simulink model "PF_ToolwithMedusa_Fix"  (R2016a)
settings: Solver=ode45  StartTime=0.0  StopTime=250  FixedStep=Ts  RelTol=1e-3
values from neighbouring files (symbols this model uses):
  Ts = 0.2    [PFtools.m]    (also in RK4_integrator.m = input.Ts; Trajectory_tracking.m = 0.1)
settings Model: Creator=hung  LastModifiedBy=hung
settings DataIOCC: LimitDataPoints=on  SaveFormat=Array
settings DebuggingCC: UnderspecifiedInitializationDetection=Classic  MergeDetectMultiDrivingBlocksExec=none  SolverPrmCheckMsg=warning  StateNameClashWarn=warning
settings HardwareCC: ProdBitPerPointer=32  ProdLargestAtomicFloat=None  ProdIntDivRoundTo=Undefined  ProdEndianess=Unspecified  ProdWordSize=32  ProdHWDeviceType=32-bit Generic
settings ModelReferenceCC: PropagateSignalLabelsOutOfModel=off
settings ConfigComp: CovModelRefEnable=Off

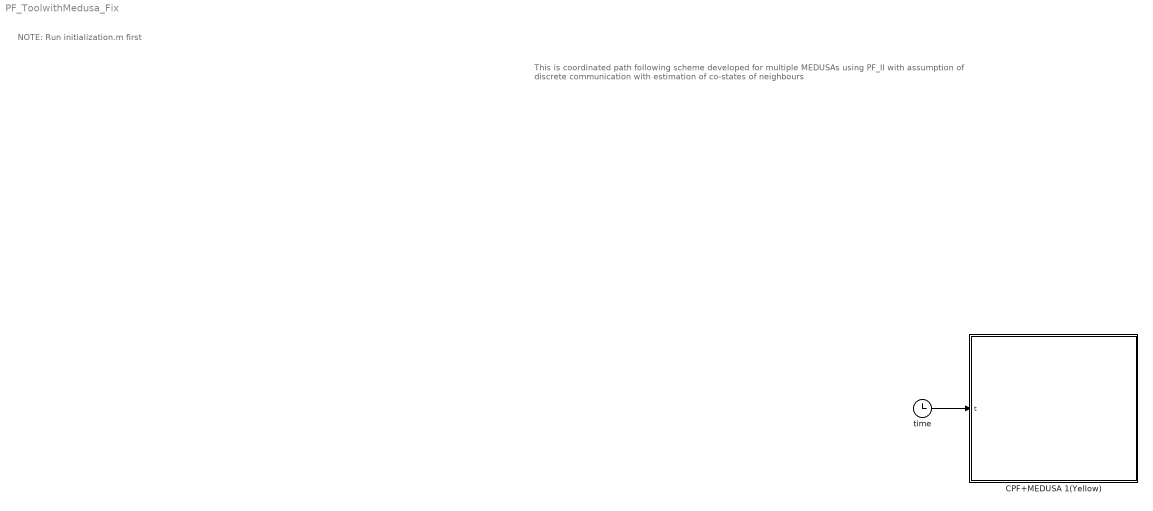
== system PF_ToolwithMedusa_Fix ==
  note: NOTE: Run initialization.m first
  note: This is coordinated path following scheme developed for multiple MEDUSAs using PF_II with
      | assumption of discrete communication with estimation of co-states of neighbours
  CPF+MEDUSA 1(Yellow) : Subsystem  Priority=2  TreatAsAtomicUnit=on  mask{Vehicle_Index=1}
      mask Display: image('MEDUSA_YELLOW.png');
  time : Clock
  wires:
  time/1 -> CPF+MEDUSA 1(Yellow)/1(t)

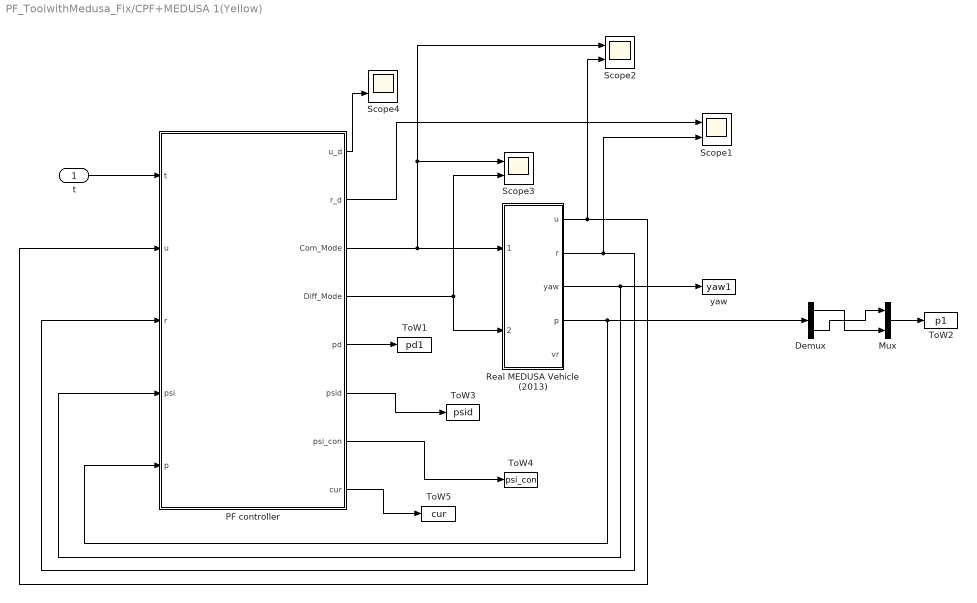
== system PF_ToolwithMedusa_Fix/CPF+MEDUSA 1(Yellow) ==
  t : Inport
  " Real MEDUSA Vehicle (2013)" : Subsystem  AncestorBlock=|
      | Mylibrary/
      | Real MEDUSA Vehicle (2013)
  Demux : Demux  Outputs=2
  Mux : Mux  Inputs=2
  "PF controller " : MATLAB Function  TreatAsAtomicUnit=on
  Scope{1..4} (4 alike) : Scope  NumInputPorts=2
  ToW1 : ToWorkspace  VariableName=pd1  SampleTime=Ts
      settings: Save2DSignal=2-D array (concatenate along first dimension)
  ToW2 : ToWorkspace  VariableName=p1  SampleTime=Ts
  ToW3 : ToWorkspace  VariableName=psid  SampleTime=Ts
      settings: Save2DSignal=2-D array (concatenate along first dimension)
  ToW4 : ToWorkspace  VariableName=psi_con  SampleTime=Ts
      settings: Save2DSignal=2-D array (concatenate along first dimension)
  ToW5 : ToWorkspace  VariableName=cur  SampleTime=Ts
      settings: Save2DSignal=2-D array (concatenate along first dimension)
  yaw : ToWorkspace  VariableName=yaw1  SampleTime=Ts
  wires:
  t/1 -> "PF controller "/1(t)
  "PF controller "/5(pd) -> ToW1/1
  "PF controller "/3(Com_Mode) -> " Real MEDUSA Vehicle (2013)"/1(Com Mode), Scope2/1, Scope3/1
  "PF controller "/2(r_d) -> Scope1/1
  "PF controller "/4(Diff_Mode) -> " Real MEDUSA Vehicle (2013)"/2(Diff Mode), Scope3/2
  " Real MEDUSA Vehicle (2013)"/4(p) -> Demux/1, "PF controller "/5(p)
  " Real MEDUSA Vehicle (2013)"/3(yaw) -> yaw/1, "PF controller "/4(psi)
  " Real MEDUSA Vehicle (2013)"/2(r) -> Scope1/2, "PF controller "/3(r)
  " Real MEDUSA Vehicle (2013)"/1(u) -> Scope2/2, "PF controller "/2(u)
  "PF controller "/6(psid) -> ToW3/1
  "PF controller "/7(psi_con) -> ToW4/1
  Mux/1 -> ToW2/1
  "PF controller "/8(cur) -> ToW5/1
  Demux/1 -> Mux/2
  Demux/2 -> Mux/1
  "PF controller "/1(u_d) -> Scope4/2

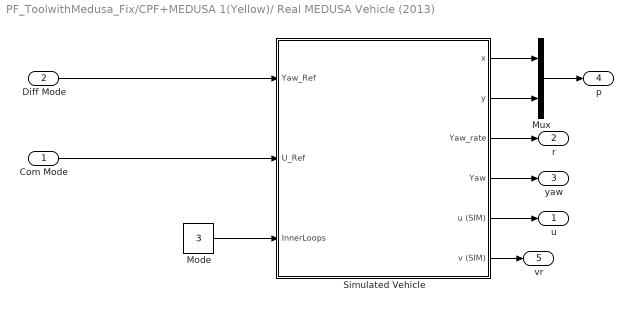
== system PF_ToolwithMedusa_Fix/CPF+MEDUSA 1(Yellow)/ Real MEDUSA Vehicle (2013) ==
  Com Mode : Inport
  Diff Mode : Inport  Port=2
  Mode : Constant  Value=3
  Mux : Mux  Inputs=2
  Simulated Vehicle : Subsystem
  u : Outport
  r : Outport  Port=2
  yaw : Outport  Port=3
  p : Outport  Port=4
  vr : Outport  Port=5
  wires:
  Diff Mode/1 -> Simulated Vehicle/1(Yaw_Ref)
  Com Mode/1 -> Simulated Vehicle/2(U_Ref)
  Mode/1 -> Simulated Vehicle/3(InnerLoops)
  Mux/1 -> p/1
  Simulated Vehicle/5(u (SIM)) -> u/1
  Simulated Vehicle/6(v (SIM)) -> vr/1
  Simulated Vehicle/3(Yaw_rate) -> r/1
  Simulated Vehicle/4(Yaw) -> yaw/1
  Simulated Vehicle/1(x) -> Mux/1
  Simulated Vehicle/2(y) -> Mux/2

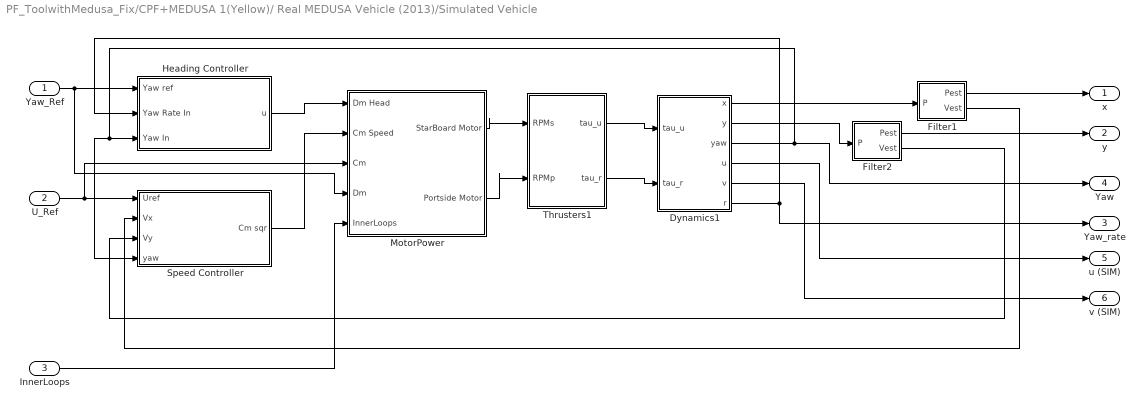
== system PF_ToolwithMedusa_Fix/CPF+MEDUSA 1(Yellow)/ Real MEDUSA Vehicle (2013)/Simulated Vehicle ==
  Yaw_Ref : Inport
  U_Ref : Inport  Port=2
  InnerLoops : Inport  Port=3
  Dynamics1 : Subsystem  mask{x0=200, y0=305, yaw0=pi/2, u0=0, v0=0, r0=0, dist_u=0, dist_v=0, dist_r=0, Vcx=0, Vcy=0}
      mask prompts: dist_u "Disturbance in u"; dist_v "Disturbance in v"; dist_r "Disturbance in r"; Vcx "Current x"; Vcy "Current y"
  Filter1 : Subsystem
  Filter2 : Subsystem
  Heading Controller : Subsystem  mask{Kp=45, Kd=110}
  MotorPower : Subsystem
  "Speed Controller " : Subsystem  mask{Kpu=60, Kiu=2, KSat=60}
      mask prompts: Kpu "Kp"; Kiu "Ki"; KSat "Common Mode Saturation"
  Thrusters1 : Subsystem
  x : Outport
  y : Outport  Port=2
  Yaw_rate : Outport  Port=3
  Yaw : Outport  Port=4
  u (SIM) : Outport  Port=5
  v (SIM) : Outport  Port=6
  wires:
  Thrusters1/1(tau_u) -> Dynamics1/1(tau_u)
  Thrusters1/2(tau_r) -> Dynamics1/2(tau_r)
  Dynamics1/1(x) -> Filter1/1(P)
  Dynamics1/2(y) -> Filter2/1(P)
  Dynamics1/3(yaw) -> Heading Controller/3(Yaw In), "Speed Controller "/4(yaw), Yaw/1
  MotorPower/1(StarBoard Motor) -> Thrusters1/1(RPMs)
  MotorPower/2(Portside Motor) -> Thrusters1/2(RPMp)
  Dynamics1/6(r) -> Heading Controller/2(Yaw Rate In), Yaw_rate/1
  Filter1/2(Vest) -> "Speed Controller "/2(Vx)
  Filter2/2(Vest) -> "Speed Controller "/3(Vy)
  "Speed Controller "/1(Cm sqr) -> MotorPower/2(Cm Speed)
  Yaw_Ref/1 -> Heading Controller/1(Yaw ref), MotorPower/4(Dm)
  Filter1/1(Pest) -> x/1
  Filter2/1(Pest) -> y/1
  U_Ref/1 -> "Speed Controller "/1(Uref), MotorPower/3(Cm)
  Heading Controller/1(u) -> MotorPower/1(Dm Head)
  InnerLoops/1 -> MotorPower/5(InnerLoops)
  Dynamics1/4(u) -> u (SIM)/1
  Dynamics1/5(v) -> v (SIM)/1

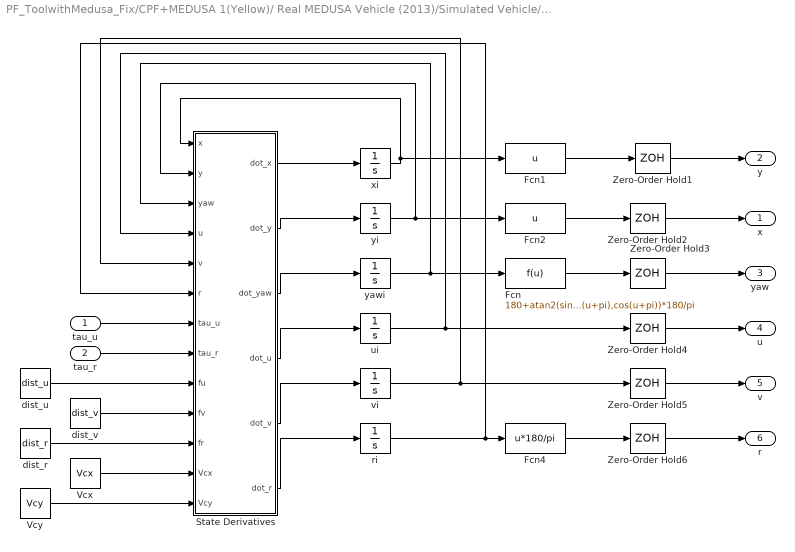
== system PF_ToolwithMedusa_Fix/CPF+MEDUSA 1(Yellow)/ Real MEDUSA Vehicle (2013)/Simulated Vehicle/Dynamics1 ==
  tau_u : Inport
  tau_r : Inport  Port=2
  Fcn : Fcn  Expr=180+atan2(sin(u+pi),cos(u+pi))*180/pi
  Fcn1 : Fcn  Expr=u
  Fcn2 : Fcn  Expr=u
  Fcn4 : Fcn  Expr=u*180/pi
  State Derivatives : MATLAB Function  TreatAsAtomicUnit=on
  Vcx : Constant  Value=Vcx
  Vcy : Constant  Value=Vcy
  Zero-Order Hold{1..6} (6 alike) : ZeroOrderHold  SampleTime=0.2
  dist_r : Constant  Value=dist_r
  dist_u : Constant  Value=dist_u
  dist_v : Constant  Value=dist_v
  ri : Integrator  InitialCondition=r0
  ui : Integrator  InitialCondition=u0
  vi : Integrator  InitialCondition=v0
  xi : Integrator  InitialCondition=y0
  yawi : Integrator  InitialCondition=yaw0
  yi : Integrator  InitialCondition=x0
  x : Outport
  y : Outport  Port=2
  yaw : Outport  Port=3
  u : Outport  Port=4
  v : Outport  Port=5
  r : Outport  Port=6
  wires:
  Fcn4/1 -> Zero-Order Hold6/1
  State Derivatives/1(dot_x) -> xi/1
  State Derivatives/2(dot_y) -> yi/1
  State Derivatives/3(dot_yaw) -> yawi/1
  State Derivatives/4(dot_u) -> ui/1
  State Derivatives/5(dot_v) -> vi/1
  State Derivatives/6(dot_r) -> ri/1
  tau_u/1 -> State Derivatives/7(tau_u)
  yi/1 -> State Derivatives/2(y), Fcn2/1
  xi/1 -> State Derivatives/1(x), Fcn1/1
  yawi/1 -> Fcn/1, State Derivatives/3(yaw)
  ui/1 -> State Derivatives/4(u), Zero-Order Hold4/1
  ri/1 -> Fcn4/1, State Derivatives/6(r)
  vi/1 -> State Derivatives/5(v), Zero-Order Hold5/1
  tau_r/1 -> State Derivatives/8(tau_r)
  dist_u/1 -> State Derivatives/9(fu)
  dist_v/1 -> State Derivatives/10(fv)
  dist_r/1 -> State Derivatives/11(fr)
  Fcn/1 -> Zero-Order Hold3/1
  Vcx/1 -> State Derivatives/12(Vcx)
  Vcy/1 -> State Derivatives/13(Vcy)
  Fcn1/1 -> Zero-Order Hold1/1
  Fcn2/1 -> Zero-Order Hold2/1
  Zero-Order Hold1/1 -> y/1
  Zero-Order Hold2/1 -> x/1
  Zero-Order Hold3/1 -> yaw/1
  Zero-Order Hold4/1 -> u/1
  Zero-Order Hold5/1 -> v/1
  Zero-Order Hold6/1 -> r/1

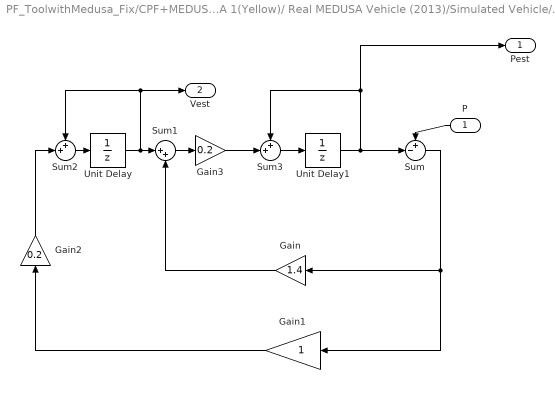
== system PF_ToolwithMedusa_Fix/CPF+MEDUSA 1(Yellow)/ Real MEDUSA Vehicle (2013)/Simulated Vehicle/Filter1 ==
  P : Inport
  Gain : Gain  Gain=1.4
  Gain1 : Gain
  Gain2 : Gain  Gain=0.2
  Gain3 : Gain  Gain=0.2
  Sum : Sum  Inputs=+-|
  Sum1 : Sum  Inputs=|++
  Sum2 : Sum  Inputs=++|
  Sum3 : Sum  Inputs=++|
  Unit Delay : UnitDelay  SampleTime=-1
  Unit Delay1 : UnitDelay  InitialCondition=200  SampleTime=-1
  Pest : Outport
  Vest : Outport  Port=2
  wires:
  Sum3/1 -> Unit Delay1/1
  Unit Delay1/1 -> Pest/1, Sum3/1, Sum/2
  Gain3/1 -> Sum3/2
  Gain2/1 -> Sum2/2
  Sum2/1 -> Unit Delay/1
  P/1 -> Sum/1
  Gain1/1 -> Gain2/1
  Unit Delay/1 -> Vest/1, Sum2/1, Sum1/1
  Gain/1 -> Sum1/2
  Sum/1 -> Gain1/1, Gain/1
  Sum1/1 -> Gain3/1

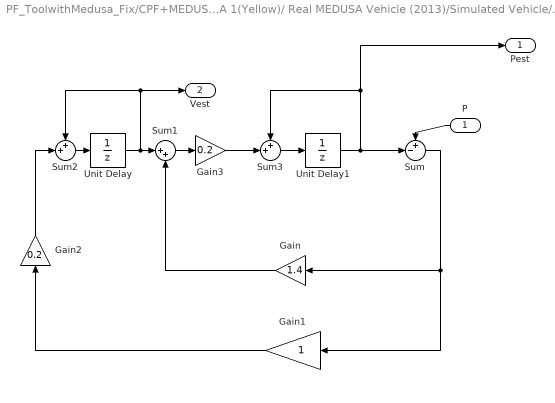
== system PF_ToolwithMedusa_Fix/CPF+MEDUSA 1(Yellow)/ Real MEDUSA Vehicle (2013)/Simulated Vehicle/Filter2 ==
  P : Inport
  Gain : Gain  Gain=1.4
  Gain1 : Gain
  Gain2 : Gain  Gain=0.2
  Gain3 : Gain  Gain=0.2
  Sum : Sum  Inputs=+-|
  Sum1 : Sum  Inputs=|++
  Sum2 : Sum  Inputs=++|
  Sum3 : Sum  Inputs=++|
  Unit Delay : UnitDelay  SampleTime=-1
  Unit Delay1 : UnitDelay  InitialCondition=305  SampleTime=-1
  Pest : Outport
  Vest : Outport  Port=2
  wires:
  Sum1/1 -> Gain3/1
  Sum/1 -> Gain/1, Gain1/1
  Gain/1 -> Sum1/2
  Unit Delay/1 -> Sum1/1, Sum2/1, Vest/1
  Gain1/1 -> Gain2/1
  P/1 -> Sum/1
  Sum2/1 -> Unit Delay/1
  Gain2/1 -> Sum2/2
  Gain3/1 -> Sum3/2
  Unit Delay1/1 -> Sum/2, Sum3/1, Pest/1
  Sum3/1 -> Unit Delay1/1

== system PF_ToolwithMedusa_Fix/CPF+MEDUSA 1(Yellow)/ Real MEDUSA Vehicle (2013)/Simulated Vehicle/Heading Controller ==
  note: 0-360
  note: Saida em Percentagem
  Yaw ref : Inport  SampleTime=Ts
  Yaw Rate In : Inport  Port=2  SampleTime=Ts
  Yaw In : Inport  Port=3
  Embedded MATLAB Function1 : MATLAB Function  TreatAsAtomicUnit=on
  sat : Saturate  UpperLimit=Inf  LowerLimit=-Inf  SampleTime=Ts
  u : Outport
  wires:
  Yaw ref/1 -> Embedded MATLAB Function1/1(YawRef)
  Embedded MATLAB Function1/1(x) -> sat/1
  Yaw In/1 -> Embedded MATLAB Function1/2(Yaw)
  Yaw Rate In/1 -> Embedded MATLAB Function1/3(Yawrate)
  sat/1 -> u/1

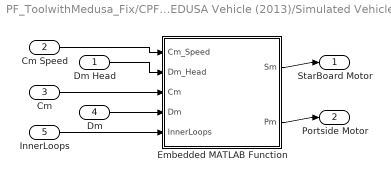
== system PF_ToolwithMedusa_Fix/CPF+MEDUSA 1(Yellow)/ Real MEDUSA Vehicle (2013)/Simulated Vehicle/MotorPower ==
  Dm Head : Inport
  Cm Speed : Inport  Port=2
  Cm : Inport  Port=3
  Dm : Inport  Port=4
  InnerLoops : Inport  Port=5
  Embedded MATLAB Function : MATLAB Function  TreatAsAtomicUnit=on
  StarBoard Motor : Outport
  Portside Motor : Outport  Port=2
  wires:
  Embedded MATLAB Function/2(Pm) -> Portside Motor/1
  Embedded MATLAB Function/1(Sm) -> StarBoard Motor/1
  Dm Head/1 -> Embedded MATLAB Function/2(Dm_Head)
  Cm Speed/1 -> Embedded MATLAB Function/1(Cm_Speed)
  Cm/1 -> Embedded MATLAB Function/3(Cm)
  Dm/1 -> Embedded MATLAB Function/4(Dm)
  InnerLoops/1 -> Embedded MATLAB Function/5(InnerLoops)

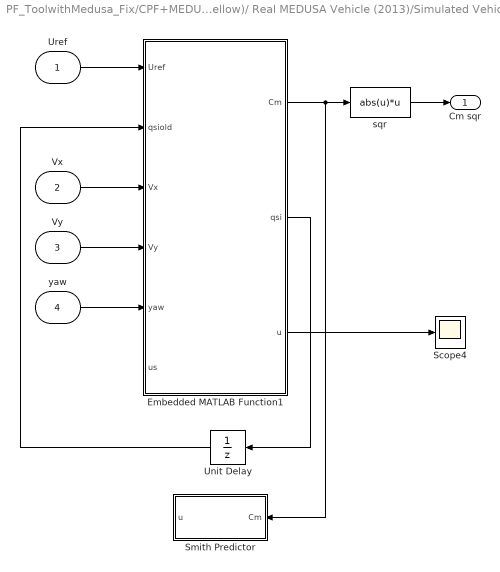
== system PF_ToolwithMedusa_Fix/CPF+MEDUSA 1(Yellow)/ Real MEDUSA Vehicle (2013)/Simulated Vehicle/Speed Controller  ==
  Uref : Inport
  Vx : Inport  Port=2
  Vy : Inport  Port=3
  yaw : Inport  Port=4
  Embedded MATLAB Function1 : MATLAB Function  TreatAsAtomicUnit=on
  Scope4 : Scope
  Smith Predictor : Subsystem
  Unit Delay : UnitDelay  SampleTime=0.2
  sqr : Fcn  Expr=abs(u)*u
  Cm sqr : Outport
  wires:
  Embedded MATLAB Function1/3(u) -> Scope4/1
  yaw/1 -> Embedded MATLAB Function1/5(yaw)
  Vy/1 -> Embedded MATLAB Function1/4(Vy)
  Vx/1 -> Embedded MATLAB Function1/3(Vx)
  Embedded MATLAB Function1/1(Cm) -> Smith Predictor/1(Cm), sqr/1
  Uref/1 -> Embedded MATLAB Function1/1(Uref)
  Embedded MATLAB Function1/2(qsi) -> Unit Delay/1
  Unit Delay/1 -> Embedded MATLAB Function1/2(qsiold)
  sqr/1 -> Cm sqr/1

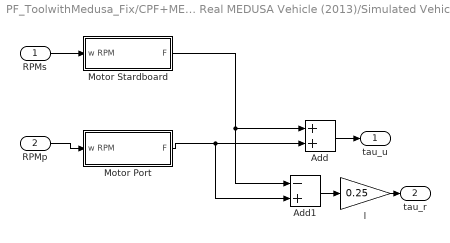
== system PF_ToolwithMedusa_Fix/CPF+MEDUSA 1(Yellow)/ Real MEDUSA Vehicle (2013)/Simulated Vehicle/Thrusters1 ==
  RPMs : Inport
  RPMp : Inport  Port=2
  Add : Sum
  Add1 : Sum  Inputs=-+
  Motor Port : Subsystem  mask{K0=7.2115, tau=0.346, eta=4/(1500^2)}
      mask prompts: tau "Atraso do Motor"; eta "Constante de conversao W-F"
  Motor Stardboard : Subsystem  mask{K0=7.2115, tau=0.346, eta=4/(1500^2)}
      mask prompts: tau "Atraso do Motor"; eta "Constante de conversao W-F"
  l : Gain  Gain=0.25
  tau_u : Outport
  tau_r : Outport  Port=2
  wires:
  Add1/1 -> l/1
  RPMs/1 -> Motor Stardboard/1(w RPM)
  Add/1 -> tau_u/1
  RPMp/1 -> Motor Port/1(w RPM)
  l/1 -> tau_r/1
  Motor Port/1(F) -> Add/2, Add1/2
  Motor Stardboard/1(F) -> Add/1, Add1/1

== system PF_ToolwithMedusa_Fix/CPF+MEDUSA 1(Yellow)/ Real MEDUSA Vehicle (2013)/Simulated Vehicle/Speed Controller /Smith Predictor ==
  Cm : Inport
  Common mode to u : DiscreteTransferFcn  Numerator=[0.0006641 0]  Denominator=[1 -0.6368 -0.2936]  SampleTime=0.2
  Integer Delay2 : Delay  DelayLength=7  InputProcessing=Inherited  SampleTime=0.2
  Sum2 : Sum  Inputs=|-+
  u : Outport
  wires:
  Cm/1 -> Common mode to u/1
  Common mode to u/1 -> Integer Delay2/1, Sum2/2
  Integer Delay2/1 -> Sum2/1
  Sum2/1 -> u/1

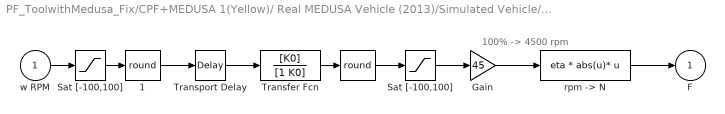
== system PF_ToolwithMedusa_Fix/CPF+MEDUSA 1(Yellow)/ Real MEDUSA Vehicle (2013)/Simulated Vehicle/Thrusters1/Motor Port ==
  note: 100% -> 4500 rpm
  w RPM : Inport
  "  " : Rounding  Operator=round
  "  1" : Rounding  Operator=round
  Gain : Gain  Gain=45
  Sat [-100,100] : Saturate  UpperLimit=100  LowerLimit=-100
  "Sat [-100,100] " : Saturate  UpperLimit=100  LowerLimit=-100
  Transfer Fcn : TransferFcn  Numerator=[K0]  Denominator=[1 K0]
  Transport Delay : TransportDelay  DelayTime=tau
  "rpm -> N" : Fcn  Expr=eta * abs(u)* u
  F : Outport
  wires:
  Transfer Fcn/1 -> "  "/1
  Transport Delay/1 -> Transfer Fcn/1
  "  1"/1 -> Transport Delay/1
  "  "/1 -> "Sat [-100,100] "/1
  "rpm -> N"/1 -> F/1
  Sat [-100,100]/1 -> "  1"/1
  Gain/1 -> "rpm -> N"/1
  w RPM/1 -> Sat [-100,100]/1
  "Sat [-100,100] "/1 -> Gain/1

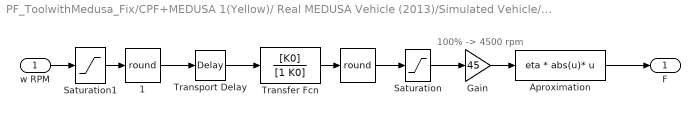
== system PF_ToolwithMedusa_Fix/CPF+MEDUSA 1(Yellow)/ Real MEDUSA Vehicle (2013)/Simulated Vehicle/Thrusters1/Motor Stardboard ==
  note: 100% -> 4500 rpm
  w RPM : Inport
  "  " : Rounding  Operator=round
  "  1" : Rounding  Operator=round
  Aproximation : Fcn  Expr=eta * abs(u)* u
  Gain : Gain  Gain=45
  Saturation : Saturate  UpperLimit=100  LowerLimit=-100
  Saturation1 : Saturate  UpperLimit=100  LowerLimit=-100
  Transfer Fcn : TransferFcn  Numerator=[K0]  Denominator=[1 K0]
  Transport Delay : TransportDelay  DelayTime=tau
  F : Outport
  wires:
  Transfer Fcn/1 -> "  "/1
  Transport Delay/1 -> Transfer Fcn/1
  "  1"/1 -> Transport Delay/1
  "  "/1 -> Saturation/1
  Aproximation/1 -> F/1
  Saturation1/1 -> "  1"/1
  Gain/1 -> Aproximation/1
  w RPM/1 -> Saturation1/1
  Saturation/1 -> Gain/1

== matlab function PF_ToolwithMedusa_Fix/CPF+MEDUSA 1(Yellow)/ Real MEDUSA Vehicle (2013)/Simulated Vehicle/Heading Controller/Embedded MATLAB Function1 ==
  data: YawRef input; x output; Yaw input; Yawrate input; Kd parameter; Kp parameter
function x = controller(YawRef, Yaw, Yawrate, Kd, Kp)
err = ( YawRef- Yaw );
if(err>180) 
     err=err-360;
elseif(err<-180) 
     err=360+err;
end

x=Kp*err-Kd*Yawrate;

== matlab function PF_ToolwithMedusa_Fix/CPF+MEDUSA 1(Yellow)/ Real MEDUSA Vehicle (2013)/Simulated Vehicle/MotorPower/Embedded MATLAB Function ==
  data: Sm output; Pm output; Cm_Speed input; Dm_Head input; Cm input; Dm input; InnerLoops input
function [Sm,Pm] = fcn(Cm_Speed, Dm_Head, Cm, Dm, InnerLoops)
Cm_sqr=0;
Dm_sqr=0;
switch InnerLoops
    case 0
        ; % Don't do anything
    case 1
        Cm_sqr=Cm_Speed;
        Dm_sqr=Dm_Head;
    case 2
        Cm_sqr=Cm*abs(Cm);
        Dm_sqr=Dm_Head;
    case 3
        Cm_sqr=Cm_Speed;
        Dm_sqr=Dm*abs(Dm);
    case 4
        Cm_sqr=Cm*abs(Cm);
        Dm_sqr=Dm*abs(Dm);
    otherwise
end

Pm = round(sqrt(abs(Cm_sqr+Dm_sqr))*sign(Cm_sqr+Dm_sqr));
Sm = round(sqrt(abs(Cm_sqr-Dm_sqr))*sign(Cm_sqr-Dm_sqr));

== matlab function PF_ToolwithMedusa_Fix/CPF+MEDUSA 1(Yellow)/ Real MEDUSA Vehicle (2013)/Simulated Vehicle/Speed Controller /Embedded MATLAB Function1 ==
  data: Cm output; Uref input; Kpu parameter; Kiu parameter; qsiold input; qsi output; Vx input; Vy input; yaw input; u output; us input; KSat parameter
function [Cm, qsi, u] = controller(Uref, Kpu,Kiu, qsiold,Vx,Vy,yaw, us, KSat)
u=Vx*sind(yaw)+Vy*cosd(yaw);
err=u-Uref;
qsi=qsiold+err;

Cm=-Kpu*(err+us)-Kiu*qsi;
% Cm =+40*Uref-Kiu*qsi;
% if(t>10)
%     qsi=qsiold+err;
%     Cm =-Kpu*err-Kiu*qsi;
% end
if(abs(Cm) >= KSat)
   Cm = KSat*sign(Cm); 
   qsi = qsiold;
end

== matlab function PF_ToolwithMedusa_Fix/CPF+MEDUSA 1(Yellow)/ Real MEDUSA Vehicle (2013)/Simulated Vehicle/Dynamics1/State Derivatives ==
  data: x input; y input; yaw input; u input; v input; r input; tau_u input; dot_x output; tau_r input; dot_y output; dot_yaw output; dot_u output; dot_v output; dot_r output; fu input; fv input; fr input; Vcx input; Vcy input
function [dot_x,dot_y,dot_yaw,dot_u,dot_v,dot_r] = fcn(x,y,yaw,u,v,r,tau_u,tau_r,fu,fv,fr, Vcx, Vcy)
%state = [x, y, yaw, u, v, r]

% %%%%%% Coefficients
% mass = 17.0;
% I_z = 4.14;
% X_dot_u = -20;
% Y_dot_v = -1.3175;
% N_dot_r =  -8.69;
% X_u = -0.2;
% Y_v = -55.117;
% N_r = -4.14;
% X_uu = -25; 
% Y_vv = -101.2776;
% N_rr = -6.23;

%%%%%% Coefficients
mass = 17.0;
I_z = 1;
X_dot_u = -20;
Y_dot_v = -30;%-1.3175;
N_dot_r = -8.69;% -0.5;
X_u = -0.2;
Y_v = -50;
N_r = -4.14; %-0.1
X_uu = -25; 
Y_vv = -0.01;%-101.2776;
N_rr = -6.23; %-21

%%%%%% masses
m_u = mass - X_dot_u;
m_v = mass - Y_dot_v;
m_r = I_z - N_dot_r;
m_uv = m_u - m_v;

%%%%%%%%% drag

d_u = -X_u - X_uu*abs(u);
d_v = -Y_v - Y_vv*abs(v);
d_r = -N_r - N_rr*abs(r);

%%%%%%%%% Dynamics

dot_u = 1/m_u*(tau_u + m_v*v*r - d_u*u+fu);
dot_v = 1/m_v*(-m_u*u*r - d_v*v+fv);
dot_r = 1/m_r*(tau_r + m_uv*u*v - d_r*r+fr);

dot_x = u*cos(yaw) - v*sin(yaw) + Vcx;
dot_y = u*sin(yaw) + v*cos(yaw) + Vcy;
dot_yaw = r;

== matlab function PF_ToolwithMedusa_Fix/CPF+MEDUSA 1(Yellow)/PF controller  ==
  settings: updateMethod=DISCRETE  sampleTime=0.2
  data: t input size=1; u input size=1; r input size=1; psi input size=1; p input size=2; u_d output size=1; r_d output size=1; Com_Mode output size=1; Diff_Mode output size=1; pd output size=2; psid output; psi_con output; cur output
%% Path following controller
% u: linear speed, % r: yaw_rate, 
% p: position, psi: yaw, 
function [u_d,r_d,Com_Mode,Diff_Mode,pd,psid,psi_con,cur] = MainPF(t,u,r,psi,p)             
%% Make all variable consistent in coordinates
p=p([2 1]);                                                                % swap x-y
psi=psi*pi/180;                                                            % convert to radian 
%% Declare variables
Ts=0.2;                                                                    % sampling time
persistent gamma PathSegment
persistent psi_old psi_con_old;
if isempty (gamma)
   gamma=0;        
   PathSegment=1;
   psi_old=psi;
   psi_con_old=psi;
end
%% Step 1: Update the current estimation in Innertial frame
% Vc_hat=CurrentEstimate(p,psi,u);                                           % in body frame
Vc_hat=[0;0];
%% Step 2: Update the path 
x_path=polypath(gamma,PathSegment);
pd=x_path(1:2);
psid=x_path(3);
cur=x_path;
% x_path=lawnpath(gamma,PathSegment);
%% Step 3: Call Path following Controller
psi_con=convert(psi,psi_old, psi_con_old);                                 % to make yaw continous from -infinity to infinity
psi_old=psi;
psi_con_old=psi_con;
vd=0.5;                                                                    % Set norminal speed of vehicle
ControllerType='Aguiar';                                                     % Hung or Lapierre or Aguiar
upf=PFcontrollers(p,psi_con,x_path,ControllerType,vd,Ts,Vc_hat,u);
%% Step 4: Call Inner loop to compute Com_Mode and Diff_Mode
 u_d=upf(1); r_d=upf(2)*180/pi;  
%   Com_Mode=SpeedController(u_d,u,Ts) ;                                     % use SpeedController of Hung. innerloop Mode=4
 Com_Mode=u_d;                                                             % use speed controller of Jorge,  innnerloop Mode=3
 Diff_Mode=YawRateController(r_d,r,Ts);
% Com_Mode=20; Diff_Mode=0;
%% Step 5: Update gamma and segment of the path 
 gammadot=upf(3); 
 % gammadot=0.01;
 gamma=gamma+Ts*gammadot;                                                   % use simple Euler integrator, we can use RK4 integrator to get better result  
%  gamma=rk4_step(@gamma_dynamics,gamma,gammadot,Ts/4);    
    if gamma >=1                                                           % this only applied for polynominal path of Sir Quintas    
        gamma=0;                                                           % reset gamma
        PathSegment=PathSegment+1;
    end   
    if PathSegment > 6
        Com_Mode=0;Diff_Mode=0;
        u_d=0; r_d=0;
        pd=[0;0];
    end
end
 
%% Polynominal path
function x_path=polypath(gamma,PathSegment)
A= [300;-22.0831438439972;-48.3661922083384;43.2340643760851;272.784728323750;10.1850969333362;62.4563880921724;-38.8628596856161;306.563353663642;20.8736774665186;-39.3413304622351;24.5089562405296;312.604656908455;13.4109050451431;23.1330811457404;-15.7093098606661;333.439333238673;18.8014159371509;-116.194384864521;101.979172953604;338.025537264906;39.0084468699079;61.9167358358428;-38.9507199706570];
B=[200;11.1792994631689;7.43748511181482;3.34062165305735;221.957406228041;33.7512849728170;-28.8604539084364;16.1098051162482;242.958042408670;27.4715205357390;32.5352997466514;-20.4656688689046;282.499193822156;26.5738139527805;-17.1347376726829;12.0438239860658;303.982094088319;42.6032060853750;108.531077431015;-21.9345924489296;433.181785155780;81.8865811269234;-50.5958611132405;35.5274948305374];
i= PathSegment;  
a=  A((i-1)*4+1:(i-1)*4+4); a=[0;0;a([4 3 2 1])];
b=  B((i-1)*4+1:(i-1)*4+4); b=[0;0;b([4 3 2 1])];
    c=0;
    z=gamma+c;
    phi  =[z^5;z^4;z^3;z^2;z;1];
    dphi =[5*z^4;4*z^3;3*z^2;2*z;1];
    ddphi=[20*z^3;12*z^2;6*z;2];
    pd   =[a'*phi;b'*phi];
    xdot_gamma=a(1:5)'*dphi;     ydot_gamma=b(1:5)'*dphi;
    xddot_gamma=a(1:4)'*ddphi;   yddot_gamma=b(1:4)'*ddphi;
    pd_gamma=[xdot_gamma;ydot_gamma];
    hg=sqrt(xdot_gamma^2+ydot_gamma^2);
    cg=(xdot_gamma*yddot_gamma-ydot_gamma*xddot_gamma)/(hg^3);
    psid=atan2(ydot_gamma,xdot_gamma);
 
%      psid=atan2(xdot_gamma,ydot_gamma);
%     psid=psid*180/pi;
    % convert to make it continous
    persistent psid_old psid_con_old;
    if isempty(psid_old)
     psid_old=psid;
     psid_con_old=psid;
    end
    psid_con=convert(psid,psid_old, psid_con_old);
    psid_old=psid;
    psid_con_old=psid_con;
    x_path=[pd;psid;pd_gamma;hg;cg;gamma];
end
%% Path following controller function
function upf=PFcontrollers(p,psi,x_path,ControllerType,vd,Ts,Vc_hat,u)
persistent vd_old gammadot_old         
persistent y1_old;
if isempty(vd_old)
    vd_old=0;
    gammadot_old =0;
    y1_old=0;
end
vd_bar=0.01;
pd=x_path(1:2);
%% Compute PF error 
if strcmp(ControllerType,'Aguiar')
    pd_gamma=x_path(4:5);
    RB_I=[cos(psi)   -sin(psi);
          sin(psi)    cos(psi)]; 
    e_pf=RB_I'*(p-pd);
    delta=-1;
    Delta_inv= [1    0;
                0  -1/delta]; 
    kx=.01; ky=.05;    
    Kk=[kx 0;
        0  ky];
    ud=Delta_inv*(-Kk*tanh(e_pf-[delta;0])-Vc_hat+RB_I'*pd_gamma*vd_bar);    
    if ud(1) < 0                                                             %not allow vehicle move backward
        ud(1)= 0;
    end
    %% Gamma controller
    kz=.1; 
    vd_dot=(vd_bar-vd_old)/Ts;   
    vd_old=vd_bar;
    gammaddot=-kz*(gammadot_old-vd)+vd_dot+.01*(e_pf-[delta;0])'*RB_I'*pd_gamma; 
    gammadot=gammadot_old+Ts*gammaddot;
%     if gammadot<0;
%             gammadot=0;
%     end
    gammadot_old=gammadot;
    upf=[ud;gammadot];
else    
    psid=x_path(3);  
    hg=x_path(6);
    cg=x_path(7);
    RI_F=[cos(psid)      sin(psid);                                         % From {I} to {F}
         -sin(psid)      cos(psid)]; 
    e_f=RI_F*(p-pd);
    s1=e_f(1);
    y1=e_f(2);
    psie=psi-psid; 
    
    if strcmp(ControllerType,'Lapierre') 
        k1=.01;k2=.2;
        k3=pi/4;
        k4=.1;
        k5=.1;
        delta=-k3*tanh(k4*y1);
%        delta=0;
        u_d=vd-abs(cg);
        ydot=u_d*sin(psie)-hg*cg*gammadot_old*s1;
        %ydot=(y1-y1_old)/Ts;
         delta_dot=-k3*k4*(1-(tanh(k4*y1))^2)*ydot;
%        delta_dot=0;
        % Controller
        gammadot=(u_d*cos(psie)+k1*s1)/hg;
        if psie==delta
           r_d=delta_dot-k5*y1*u_d+cg*hg*gammadot_old;    
        else
            r_d=delta_dot-k5*y1*u_d*(sin(psie)-sin(delta))/(psie-delta)-k2*(psie-delta)+cg*hg*gammadot_old;
        end
%         if gammadot<0;
%             gammadot=0;
%         end
        y1_old=y1;
        gammadot_old=gammadot;
    elseif strcmp(ControllerType,'Hung') 
        u_d= vd-abs(cg);  
        k1=.5; k3=.28; k2=.4;
        if psie==0
            r_d=-k3*y1*u_d/(1+s1^2+y1^2)+cg*hg*gammadot_old;
        else
            r_d=-k3*y1*u_d*sin(psie)/(psie*(1+s1^2+y1^2))-k2*tanh(psie)+cg*hg*gammadot_old;
        end
        gammadot=(u_d*cos(psie)+k1*tanh(.1*s1))/hg;
        if gammadot<0;
            gammadot=0;
        end
        gammadot_old=gammadot;
    end   
    upf=[u_d;r_d;gammadot];
end
end
%% Speed controller
function Com_Mode=SpeedController(u_d,u,Ts)
 persistent eu_old Com_Mode_old Sat_C_Mode_old
 if isempty(eu_old)
     eu_old=0; Com_Mode_old=0; Sat_C_Mode_old=0;
 end
        C_max=60;  
        C_min=0; 
        eu=u_d-u;
        % Speed controller
        Kp_u=60;
        KI_u=20;
        Kd_u=0;
        Ka_u=20;
        Com_Mode=Kp_u*eu+(Ts*KI_u-Kp_u)*eu_old++Ka_u*Ts*Sat_C_Mode_old+(1-Ka_u*Ts)*Com_Mode_old;
        Sat_C_Mode=min(C_max, max(C_min, Com_Mode));
        Com_Mode_old=Com_Mode;
        eu_old=eu;
        Com_Mode=Sat_C_Mode;
end
%% Yawrate controller
function Diff_Mode=YawRateController(r_d,r,Ts)
persistent er_old Diff_Mode_old Sat_D_Mode_old
 if isempty(er_old)
     er_old=0; Diff_Mode_old=0; Sat_D_Mode_old=0;
 end
        D_max=60;  
        D_min=-60;
        er=r_d-r;
        Kp_r=4;
        KI_r=4;
        Kd_=0;
        Ka_r=4;
        Diff_Mode=Kp_r*er+(Ts*KI_r-Kp_r)*er_old+Ka_r*Ts*Sat_D_Mode_old+(1-Ka_r*Ts)*Diff_Mode_old;
        Sat_D_Mode=min(D_max, max(D_min, Diff_Mode));
        Diff_Mode_old=Diff_Mode;
        Sat_D_Mode_old=Sat_D_Mode;
        er_old=er;
        Diff_Mode=Sat_D_Mode;       
end
%% Convert Yawangle to make it continous, important in Hung and Lapier controllers
function alg_t=convert(alg,alg_old, alg_t_old)
    if (alg-alg_old>3*pi/2)
        alg_t=alg_t_old+alg-alg_old-2*pi;
    elseif (alg_old-alg>3*pi/2)
         alg_t=alg_t_old+alg-alg_old+2*pi;
    else
        alg_t=alg_t_old+alg-alg_old;
    end
end
%%%%%%%%%%%%%%%%%%%%%%%%%%%%%%%%%%%%%%%%%%%%%%%%%%%%%%%%%%%%%%%%%%%%%%%%%%%%%%%%%%%%%%%%%%%%%%%%%%%%%%%%
%            For time being, you dont need to code following functions
%%%%%%%%%%%%%%%%%%%%%%%%%%%%%%%%%%%%%%%%%%%%%%%%%%%%%%%%%%%%%%%%%%%%%%%%%%%%%%%%%%%%%%%%%%%%%%%%%%%%%%%%
%% Path function is path generator (Lawn mower)
function x_path = lawnpath(gamma,PathSegment) 
    L=50;R=12;d=0;m=0;
    s1=L-m;
    s2=s1+pi*(R-d);
    s3=s2+L;
    s4=s3+pi*(R+d);
    s5=s4+m;
    ratio1=(R-d)/R;
    ratio2=(R+d)/R;
%     ratio1=1;
%     ratio2=1;

    if gamma<s5;
        cycle=0;
    else
        cycle=1;
    end
    s=gamma-s5*cycle;
    c1=1.2/(R-d);
    c2=1/(R+d);
    k=.5;
    cur=c1/(1+exp(-k*(s-s1)))-c1/(1+exp(-k*(s-s2)))+c2/(1+exp(-k*(s-s3)))-c2/(1+exp(-k*(s-s4)));
    if s<s1                                    % first segment of straight line;
        xd=s+R+m;
        yd=0+d;
        pd_gamma=[1;0];      
    elseif (s>=s1) && (s<=s2)                  % second segment, a circumference 
        psi_T=(s-s1)/(R-d);
        xd=L+R+(R-d)*sin(psi_T);   
        yd=d+(R-d)*(1-cos(psi_T));
        pd_gamma=[cos(psi_T);sin(psi_T)]; 
    elseif (s>s2) && (s<=s3)                   % third segment, a straight line 
        xd=s3-s+R;  
        yd=d+2*(R-d); 
        pd_gamma=[-1;0];
    elseif (s>s3) && (s<=s4)   
        xd=R-(R+d)*sin((s-s3)/(R+d));
        yd=d+2*(R-d)+(R+d)*(1-cos((s-s3)/(R+d)));
        pd_gamma=[-cos((s-s3)/(R+d));sin((s-s3)/(R+d))];   
    else
        xd=(s-s4)+R;
        yd=d+4*R;
        pd_gamma=[1;0];
    end
    if cycle ==0
        pd=[xd;cycle*4*R+yd];
    else 
        pd=[xd;cycle*4*R+yd];
    end
    %% Rotate the mission
    phi=pi/4;
    R=[cos(phi)   sin(phi);
       -sin(phi)  cos(phi)]; 
    pd=R*pd;
    pd_gamma=R*pd_gamma;
    x_path=[pd;psid;pd_gamma;hg;cg;gamma];
end
%% Current estimation function
function Vc_hat=CurrentEstimate(p,yaw,ur)
    persistent p_hat_old Vcxy_hat Vcxy_hat_old p_hat p_old ur_old
    if isemty(p_hat_old)
        p_old=p;
        p_hat_old=p; p_hat=p;
        Vcxy_hat_old=[0;0]; Vcxy_hat=[0;0];
        ur_old=ur;
    end
    RB_I=[cos(yaw)        -sin(yaw);     % From {B} to {I}
          sin(yaw)         cos(yaw)]; 
    p_t=p_old-p_hat;
    Vr=[ur_old;0];
    Kp=1*[1 0;
          0 1];
    Kc=1*[1 0;
          0 1];
    p_hat_dot=RB_I*Vr+Vcxy_hat+Kp*p_t;
    p_hat=p_hat_old+Ts*p_hat_dot;
    p_hat_old=p_hat;
    Vcxy_hat_dot=Kc*p_t;
    Vcxy_hat=Vcxy_hat_old+Ts*Vcxy_hat_dot;
    Vcxy_hat_old=Vcxy_hat;
    p_old=p;
    ur_old=ur;
    Vc_hat=Vcxy_hat;
end
%% Kinematic dynamics of vehicle
 function x_next=update_vehicle(x_current,input,Ts,t)
    input_robot.nSteps = 4;
    input_robot.Ts=Ts;
    input_robot.u=input;
    input_robot.x = x_current;
    output_robot = RK4_integrator(@vehicle, input_robot);
    x_next = output_robot.value;
 end                   %% No need but for testing
%% vehicle dynamics
function dx = vehicle(t,x,u)
    psi=x(3);
    ur=u(1);
    r=u(2);
    dx=[ur*cos(psi);ur*sin(psi);r];
end                                            %% No need but for testing
%% Gamma dynamics
function dx = gamma_dynamics(t,x,u)
    dx=u;
end                                     %% No need also but for testing 
%% Runge–Kutta integrator
function x_next = rk4_step(ode_fun,x,u,h)
    k1 = ode_fun(0,x,u);
    k2 = ode_fun(0,x+h/2.*k1,u);
    k3 = ode_fun(0,x+h/2.*k2,u);
    k4 = ode_fun(0,x+h.*k3,u);
    x_next = x + h/6.*(k1+2*k2+2*k3+k4);
end                               %% No need also but for testing
